simulink model "CHEM_ATTACK_BENCHMARK_MO_3"  (R2015b)
settings: Solver=ode45  StartTime=0.0  StopTime=199.9  RelTol=1e-3
values from neighbouring files (symbols this model uses):
  A1 = 0.0154    [INIT.m]
  A2 = 0.0154    [INIT.m]
  Cvb = 1.5938*1e-4    (= 0.00015938)    [INIT.m]
  Cvo = 1.59640*1e-4    (= 0.00015964)    [INIT.m]
  h1c = 0.5    [INIT.m]
  h1c_0 = 0    [INIT.m]
  h1max = 0.6    [INIT.m]
  h2c_0 = 0.03    [INIT.m]
  h2c_max = 0.11    [INIT.m]
  h2c_min = 0.09    [INIT.m]
  h2max = 0.6    [INIT.m]
  Ki = 5*1e-6    (= 5e-06)    [INIT.m]
  Kp = 1e-3    (= 0.001)    [INIT.m]
  Qf1 = 1e-4    (= 0.0001)    [INIT.m]    (also in extract_data.m = 5e-5*randn + 1e-4)
  Qf2 = 1e-4    (= 0.0001)    [INIT.m]    (also in extract_data.m = 5e-5*randn + 1e-4)
  Qpmax = 1e-2    (= 0.01)    [INIT.m]
  rate_noise_mQp = 1e-6    (= 1e-06)    [INIT.m]
  rate_noise_mUp = 1e-6    (= 1e-06)    [INIT.m]
  rate_noise_my1 = 1e-6    (= 1e-06)    [INIT.m]
  rate_noise_my2 = 1e-6    (= 1e-06)    [INIT.m]
  Te = 1    [INIT.m]
  yo = 0    [INIT.m]
(part 5 of 5)

== system CHEM_ATTACK_BENCHMARK_MO_3/faultless/FAULTLESS FAULT/Subsystem9/Subsystem1 ==
  note: Control valve V0
  Conmmande vanne o : ManualSwitch
  closed : Constant  Value=0
  opened : Constant
  Out1 : Outport  InitialOutput=0
  wires:
  closed/1 -> Conmmande vanne o/2
  opened/1 -> Conmmande vanne o/1
  Conmmande vanne o/1 -> Out1/1

== system CHEM_ATTACK_BENCHMARK_MO_3/faultless/FAULTLESS FAULT/Subsystem9/Subsystem12 ==
  "Set of level of tank 1 " : Step  Time=0  Before=h1c_0  After=h1c  SampleTime=0
  Out1 : Outport
  wires:
  "Set of level of tank 1 "/1 -> Out1/1

== system CHEM_ATTACK_BENCHMARK_MO_3/faultless1/FAULTLESS FAULT/Subsystem9/Subsystem1 ==
  note: Control valve V0
  Conmmande vanne o : ManualSwitch
  closed : Constant  Value=0
  opened : Constant
  Out1 : Outport  InitialOutput=0
  wires:
  closed/1 -> Conmmande vanne o/2
  opened/1 -> Conmmande vanne o/1
  Conmmande vanne o/1 -> Out1/1

== system CHEM_ATTACK_BENCHMARK_MO_3/faultless1/FAULTLESS FAULT/Subsystem9/Subsystem12 ==
  "Set of level of tank 1 " : Step  Time=0  Before=h1c_0  After=h1c  SampleTime=0
  Out1 : Outport
  wires:
  "Set of level of tank 1 "/1 -> Out1/1

== system CHEM_ATTACK_BENCHMARK_MO_3/faultless2/FAULTLESS FAULT/Subsystem9/Subsystem1 ==
  note: Control valve V0
  Conmmande vanne o : ManualSwitch
  closed : Constant  Value=0
  opened : Constant
  Out1 : Outport  InitialOutput=0
  wires:
  closed/1 -> Conmmande vanne o/2
  opened/1 -> Conmmande vanne o/1
  Conmmande vanne o/1 -> Out1/1

== system CHEM_ATTACK_BENCHMARK_MO_3/faultless2/FAULTLESS FAULT/Subsystem9/Subsystem12 ==
  "Set of level of tank 1 " : Step  Time=0  Before=h1c_0  After=h1c  SampleTime=0
  Out1 : Outport
  wires:
  "Set of level of tank 1 "/1 -> Out1/1

== system CHEM_ATTACK_BENCHMARK_MO_3/faultless3/FAULTLESS FAULT/Subsystem9/Subsystem1 ==
  note: Control valve V0
  Conmmande vanne o : ManualSwitch
  closed : Constant  Value=0
  opened : Constant
  Out1 : Outport  InitialOutput=0
  wires:
  closed/1 -> Conmmande vanne o/2
  opened/1 -> Conmmande vanne o/1
  Conmmande vanne o/1 -> Out1/1

== system CHEM_ATTACK_BENCHMARK_MO_3/faultless3/FAULTLESS FAULT/Subsystem9/Subsystem12 ==
  "Set of level of tank 1 " : Step  Time=0  Before=h1c_0  After=h1c  SampleTime=0
  Out1 : Outport
  wires:
  "Set of level of tank 1 "/1 -> Out1/1

== system CHEM_ATTACK_BENCHMARK_MO_3/mUp fault/FAULTLESS FAULT/Subsystem9/Subsystem1 ==
  note: Control valve V0
  Conmmande vanne o : ManualSwitch
  closed : Constant  Value=0
  opened : Constant
  Out1 : Outport  InitialOutput=0
  wires:
  closed/1 -> Conmmande vanne o/2
  opened/1 -> Conmmande vanne o/1
  Conmmande vanne o/1 -> Out1/1

== system CHEM_ATTACK_BENCHMARK_MO_3/mUp fault/FAULTLESS FAULT/Subsystem9/Subsystem12 ==
  "Set of level of tank 1 " : Step  Time=0  Before=h1c_0  After=h1c  SampleTime=0
  Out1 : Outport
  wires:
  "Set of level of tank 1 "/1 -> Out1/1

== system CHEM_ATTACK_BENCHMARK_MO_3/my1 fault/FAULTLESS FAULT/Subsystem9/Subsystem1 ==
  note: Control valve V0
  Conmmande vanne o : ManualSwitch
  closed : Constant  Value=0
  opened : Constant
  Out1 : Outport  InitialOutput=0
  wires:
  closed/1 -> Conmmande vanne o/2
  opened/1 -> Conmmande vanne o/1
  Conmmande vanne o/1 -> Out1/1

== system CHEM_ATTACK_BENCHMARK_MO_3/my1 fault/FAULTLESS FAULT/Subsystem9/Subsystem12 ==
  "Set of level of tank 1 " : Step  Time=0  Before=h1c_0  After=h1c  SampleTime=0
  Out1 : Outport
  wires:
  "Set of level of tank 1 "/1 -> Out1/1

== system CHEM_ATTACK_BENCHMARK_MO_3/my2 fault/FAULTLESS FAULT/Subsystem9/Subsystem1 ==
  note: Control valve V0
  Conmmande vanne o : ManualSwitch
  closed : Constant  Value=0
  opened : Constant
  Out1 : Outport  InitialOutput=0
  wires:
  closed/1 -> Conmmande vanne o/2
  opened/1 -> Conmmande vanne o/1
  Conmmande vanne o/1 -> Out1/1

== system CHEM_ATTACK_BENCHMARK_MO_3/my2 fault/FAULTLESS FAULT/Subsystem9/Subsystem12 ==
  "Set of level of tank 1 " : Step  Time=0  Before=h1c_0  After=h1c  SampleTime=0
  Out1 : Outport
  wires:
  "Set of level of tank 1 "/1 -> Out1/1

== system CHEM_ATTACK_BENCHMARK_MO_3/pump fault/FAULTLESS FAULT/Subsystem9/Subsystem1 ==
  note: Control valve V0
  Conmmande vanne o : ManualSwitch
  closed : Constant  Value=0
  opened : Constant
  Out1 : Outport  InitialOutput=0
  wires:
  closed/1 -> Conmmande vanne o/2
  opened/1 -> Conmmande vanne o/1
  Conmmande vanne o/1 -> Out1/1

== system CHEM_ATTACK_BENCHMARK_MO_3/pump fault/FAULTLESS FAULT/Subsystem9/Subsystem12 ==
  "Set of level of tank 1 " : Step  Time=0  Before=h1c_0  After=h1c  SampleTime=0
  Out1 : Outport
  wires:
  "Set of level of tank 1 "/1 -> Out1/1
